simulink model "Bias_remove"  (R2022b)
settings: Solver=VariableStepAuto  StartTime=0.0  StopTime=1.1  RelTol=1e-3
values from neighbouring files (symbols this model uses):
  degs2rpm = 0.166666666667    [parameters.mat]
  der =     [parameters.mat]
  sens =     [parameters.mat]
  Ts = 0.001    [parameters.mat]
undefined symbols (not defined in the file or in its folder): bias, DiscIntNeverNeededParam, pulse2deg, simul
libraries: simulink x1
settings Model: Creator=emanuelevitetta  LastModifiedBy=emanuelevitetta

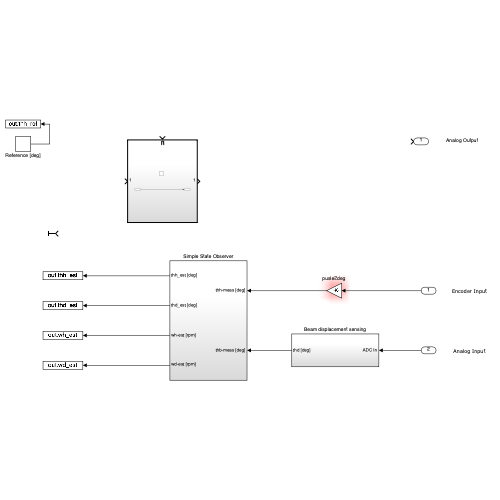
[thumbnail: Simulink's stored preview of the top-level diagram]
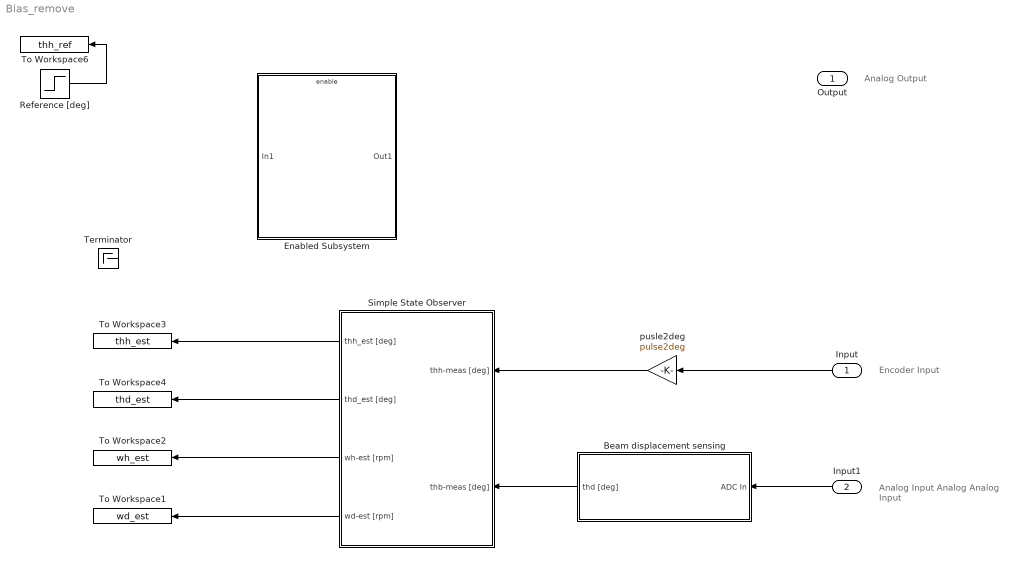
== system Bias_remove ==
  note: Encoder Input
  note: Analog Input
      |
      | Analog
      | Analog Input
  note: Analog Output
  Input : Inport
  Input1 : Inport  Port=2
  Beam displacement sensing : Subsystem
  Enabled Subsystem : Subsystem  TreatAsAtomicUnit=on
  Reference [deg] : Step  After=simul.stepdeg
  Simple State Observer : Subsystem
  Terminator : Terminator
  To Workspace1 : ToWorkspace  VariableName=wd_est  SaveFormat=Structure With Time  SampleTime=Ts
  To Workspace2 : ToWorkspace  VariableName=wh_est  SaveFormat=Structure With Time  SampleTime=Ts
  To Workspace3 : ToWorkspace  VariableName=thh_est  SaveFormat=Structure With Time  SampleTime=Ts
  To Workspace4 : ToWorkspace  VariableName=thd_est  SaveFormat=Structure With Time  SampleTime=Ts
  To Workspace6 : ToWorkspace  VariableName=thh_ref  SaveFormat=Structure With Time  SampleTime=-1
  pusle2deg : Gain  Gain=pulse2deg
  Output : Outport
  wires:
  Reference [deg]/1 -> To Workspace6/1
  Input/1 -> pusle2deg/1
  Input1/1 -> Beam displacement sensing/1(ADC In)
  Beam displacement sensing/1(thd [deg]) -> Simple State Observer/2(thb-meas [deg])
  pusle2deg/1 -> Simple State Observer/1(thh-meas [deg])
  Simple State Observer/4(wd-est [rpm]) -> To Workspace1/1
  Simple State Observer/3(wh-est [rpm]) -> To Workspace2/1
  Simple State Observer/1(thh_est [deg]) -> To Workspace3/1
  Simple State Observer/2(thd_est [deg]) -> To Workspace4/1

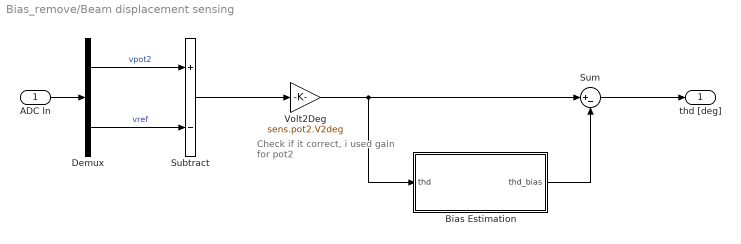
== system Bias_remove/Beam displacement sensing ==
  note: Check if it correct,
      | i used gain for pot2
  ADC In : Inport
  Bias Estimation : Subsystem
  Demux : Demux  Outputs=2
  Subtract : Sum  Inputs=+-
  Sum : Sum  Inputs=|+-
  Volt2Deg : Gain  Gain=sens.pot2.V2deg
  thd [deg] : Outport
  wires:
  ADC In/1 -> Demux/1
  Demux/1 -> Subtract/1  "vpot2"
  Demux/2 -> Subtract/2  "vref"
  Subtract/1 -> Volt2Deg/1
  Sum/1 -> thd [deg]/1
  Volt2Deg/1 -> Bias Estimation/1(thd), Sum/1
  Bias Estimation/1(thd_bias) -> Sum/2

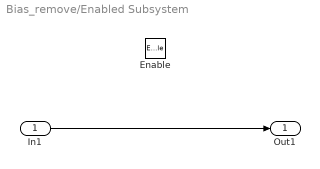
== system Bias_remove/Enabled Subsystem ==
  In1 : Inport
  Enable : EnablePort
  Out1 : Outport
  wires:
  In1/1 -> Out1/1

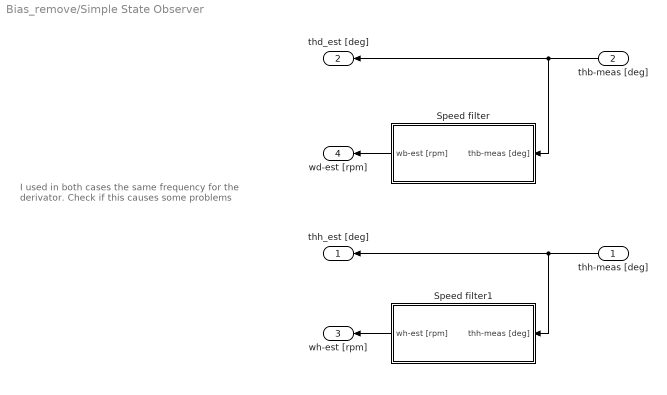
== system Bias_remove/Simple State Observer ==
  note: I used in both cases the same frequency for the derivator. Check if this causes some problems
  thh-meas [deg] : Inport
  thb-meas [deg] : Inport  Port=2
  Speed filter : Subsystem
  Speed filter1 : Subsystem
  thh_est [deg] : Outport
  thd_est [deg] : Outport  Port=2
  wh-est [rpm] : Outport  Port=3
  wd-est [rpm] : Outport  Port=4
  wires:
  thh-meas [deg]/1 -> thh_est [deg]/1, Speed filter1/1(thh-meas [deg])
  Speed filter/1(wb-est [rpm]) -> wd-est [rpm]/1
  Speed filter1/1(wh-est [rpm]) -> wh-est [rpm]/1
  thb-meas [deg]/1 -> thd_est [deg]/1, Speed filter/1(thb-meas [deg])

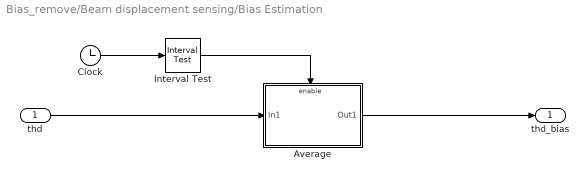
== system Bias_remove/Beam displacement sensing/Bias Estimation ==
  thd : Inport
  Average : Subsystem
  Clock : Clock
  Interval Test : simulink/Logic and Bit Operations/Interval Test  IntervalClosedRight=on  uplimit=bias.t1  IntervalClosedLeft=on  lowlimit=bias.t0  OutDataTypeStr=boolean
  thd_bias : Outport
  wires:
  Clock/1 -> Interval Test/1
  thd/1 -> Average/1(In1)
  Average/1(Out1) -> thd_bias/1
  Interval Test/1 -> Average/Enable

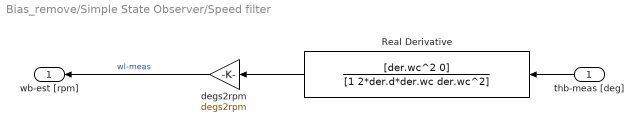
== system Bias_remove/Simple State Observer/Speed filter ==
  thb-meas [deg] : Inport
  Real Derivative : TransferFcn  Numerator=[der.wc^2 0]  Denominator=[1 2*der.d*der.wc der.wc^2]
  degs2rpm : Gain  Gain=degs2rpm
  wb-est [rpm] : Outport
  wires:
  thb-meas [deg]/1 -> Real Derivative/1
  degs2rpm/1 -> wb-est [rpm]/1  "wl-meas"
  Real Derivative/1 -> degs2rpm/1

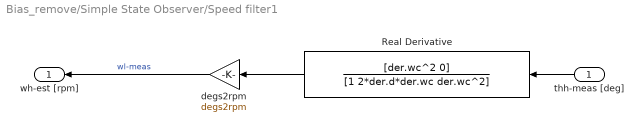
== system Bias_remove/Simple State Observer/Speed filter1 ==
  thh-meas [deg] : Inport
  Real Derivative : TransferFcn  Numerator=[der.wc^2 0]  Denominator=[1 2*der.d*der.wc der.wc^2]
  degs2rpm : Gain  Gain=degs2rpm
  wh-est [rpm] : Outport
  wires:
  thh-meas [deg]/1 -> Real Derivative/1
  degs2rpm/1 -> wh-est [rpm]/1  "wl-meas"
  Real Derivative/1 -> degs2rpm/1

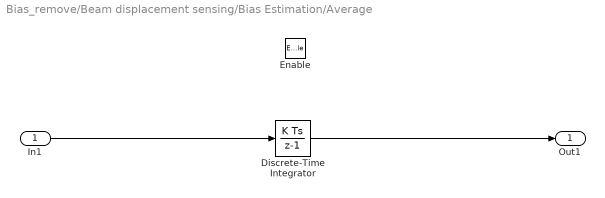
== system Bias_remove/Beam displacement sensing/Bias Estimation/Average ==
  In1 : Inport
  Enable : EnablePort
  Discrete-Time Integrator : DiscreteIntegrator  gainval=1/(bias.t1-bias.t0)  SampleTime=-1  ICPrevOutput=DiscIntNeverNeededParam  ICPrevScaledInput=DiscIntNeverNeededParam
  Out1 : Outport
  wires:
  Discrete-Time Integrator/1 -> Out1/1
  In1/1 -> Discrete-Time Integrator/1
